simulink model "Control_3_states"  (R2017b)
settings: Solver=VariableStepAuto  StartTime=0.0  StopTime=TMax  RelTol=1e-3
values from neighbouring files (symbols this model uses):
  alpha = exp(-2*pi*DT*fc)    [control_3_states.m]
  DT = 0.01    [control_3_states.m]
  G = -place(A,B,poles)    [control_3_states.m]
  PC_MaxPit = 1.570796    [control_3_states.m]
  PC_MaxRat = 0.1396263    [control_3_states.m]
  PC_MinPit = 0.0    (= 0)    [control_3_states.m]
  ref_DrTr = 0.004818    [control_3_states.m]
  ref_DrTrdot = 0    [control_3_states.m]
  ref_pitch = 7.06205E-02    (= 0.0706205)    [control_3_states.m]
  ref_rot = 1.2671090354999999    (= 1.2671090355)    [control_3_states.m]
undefined symbols (not defined in the file or in its folder): OutList, strmatch
settings Model: Creator=Avell 1513  LastModifiedBy=Avell 1513

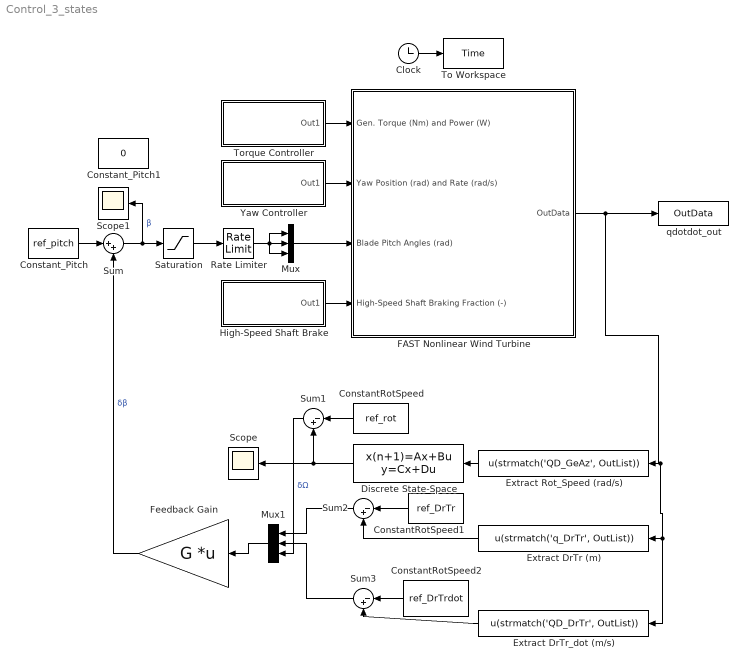
== system Control_3_states ==
  Clock : Clock
  ConstantRotSpeed : Constant  Value=ref_rot
  ConstantRotSpeed1 : Constant  Value=ref_DrTr
  ConstantRotSpeed2 : Constant  Value=ref_DrTrdot
  Constant_Pitch : Constant  Value=ref_pitch
  Constant_Pitch1 : Constant  Value=0
  Discrete State-Space : DiscreteStateSpace  A=alpha  B=1-alpha  C=alpha  D=1-alpha  InitialCondition=ref_rot  SampleTime=DT
  Extract DrTr (m) : Fcn  Expr=u(strmatch('q_DrTr', OutList))
  Extract DrTr_dot (m/s) : Fcn  Expr=u(strmatch('QD_DrTr', OutList))
  Extract Rot_Speed (rad/s) : Fcn  Expr=u(strmatch('QD_GeAz', OutList))
  FAST Nonlinear Wind Turbine : Subsystem  mask(FAST Nonlinear Wind Turbine){}
      mask help: This block contains the FAST S-Function.
      mask init:
      | clear FAST_SFunc
  Feedback Gain : Gain  Gain=G  Multiplication=Matrix(K*u)
  High-Speed Shaft Brake : Subsystem
  Mux : Mux  Inputs=3
  Mux1 : Mux  Inputs=3
  Rate Limiter : RateLimiter  RisingSlewLimit=PC_MaxRat  FallingSlewLimit=-PC_MaxRat  SampleTimeMode=inherited
  Saturation : Saturate  UpperLimit=PC_MaxPit  LowerLimit=PC_MinPit
  Scope : Scope
  Scope1 : Scope
  Sum : Sum  Inputs=|++
  Sum1 : Sum  Inputs=|-+
  Sum2 : Sum  Inputs=|-+
  Sum3 : Sum  Inputs=|-+
  To Workspace : ToWorkspace  VariableName=Time  SampleTime=-1
  Torque Controller : Subsystem
  Yaw Controller : Subsystem
  qdotdot_out : ToWorkspace  VariableName=OutData  SampleTime=-1
  wires:
  Rate Limiter/1 -> Mux/1, Mux/3, Mux/2
  Sum/1 -> Saturation/1, Scope1/1  "β"
  Torque Controller/1(Out1) -> FAST Nonlinear Wind Turbine/1(Gen. Torque (Nm) and Power (W))
  Saturation/1 -> Rate Limiter/1
  Clock/1 -> To Workspace/1
  Feedback Gain/1 -> Sum/2  "δβ"
  Discrete State-Space/1 -> Scope/1, Sum1/2
  Constant_Pitch/1 -> Sum/1
  ConstantRotSpeed/1 -> Sum1/1
  FAST Nonlinear Wind Turbine/1(OutData) -> Extract DrTr_dot (m/s)/1, Extract DrTr (m)/1, Extract Rot_Speed (rad/s)/1, qdotdot_out/1
  Yaw Controller/1(Out1) -> FAST Nonlinear Wind Turbine/2(Yaw Position (rad) and Rate (rad/s))
  Mux/1 -> FAST Nonlinear Wind Turbine/3(Blade Pitch Angles (rad))
  High-Speed Shaft Brake/1(Out1) -> FAST Nonlinear Wind Turbine/4(High-Speed Shaft Braking Fraction (-))
  Extract Rot_Speed (rad/s)/1 -> Discrete State-Space/1
  Sum1/1 -> Mux1/3  "δΩ"
  ConstantRotSpeed1/1 -> Sum2/1
  ConstantRotSpeed2/1 -> Sum3/1
  Extract DrTr (m)/1 -> Sum2/2
  Extract DrTr_dot (m/s)/1 -> Sum3/2
  Sum2/1 -> Mux1/1
  Sum3/1 -> Mux1/2
  Mux1/1 -> Feedback Gain/1

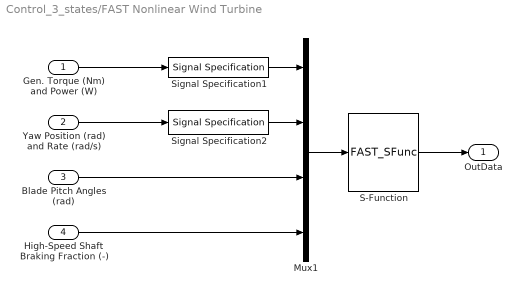
== system Control_3_states/FAST Nonlinear Wind Turbine ==
  Gen. Torque (Nm) and Power (W) : Inport
  Yaw Position (rad) and Rate (rad/s) : Inport  Port=2
  Blade Pitch Angles (rad) : Inport  Port=3
  High-Speed Shaft Braking Fraction (-) : Inport  Port=4
  Mux1 : Mux
  S-Function : S-Function  FunctionName=FAST_SFunc  Parameters=FAST_InputFileName, TMax, 0  SFunctionDeploymentMode=off  EnableBusSupport=off
  Signal Specification1 : SignalSpecification  OutDataTypeStr=double  Dimensions=2
  Signal Specification2 : SignalSpecification  OutDataTypeStr=double  Dimensions=2
  OutData : Outport
  wires:
  Gen. Torque (Nm) and Power (W)/1 -> Signal Specification1/1
  S-Function/1 -> OutData/1
  Mux1/1 -> S-Function/1
  Blade Pitch Angles (rad)/1 -> Mux1/3
  Yaw Position (rad) and Rate (rad/s)/1 -> Signal Specification2/1
  Signal Specification1/1 -> Mux1/1
  Signal Specification2/1 -> Mux1/2
  High-Speed Shaft Braking Fraction (-)/1 -> Mux1/4

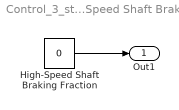
== system Control_3_states/High-Speed Shaft Brake ==
  High-Speed Shaft Braking Fraction : Constant  Value=0
  Out1 : Outport
  wires:
  High-Speed Shaft Braking Fraction/1 -> Out1/1

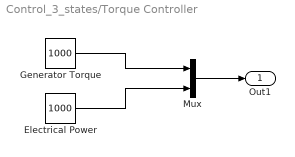
== system Control_3_states/Torque Controller ==
  Electrical Power : Constant  Value=1000
  Generator Torque : Constant  Value=1000
  Mux : Mux  Inputs=2
  Out1 : Outport
  wires:
  Mux/1 -> Out1/1
  Generator Torque/1 -> Mux/1
  Electrical Power/1 -> Mux/2

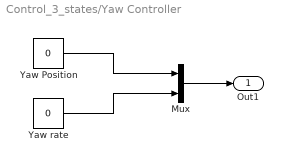
== system Control_3_states/Yaw Controller ==
  Mux : Mux  Inputs=2
  Yaw Position : Constant  Value=0
  Yaw rate : Constant  Value=0
  Out1 : Outport
  wires:
  Mux/1 -> Out1/1
  Yaw Position/1 -> Mux/1
  Yaw rate/1 -> Mux/2
